simulink model "problem2"  (R2020a)
settings: Solver=VariableStepAuto  StartTime=0.0  StopTime=10.0  RelTol=1e-3
undefined symbols (not defined in the file): be, bv, Ie, Iv, muk, mus, R
settings Model: DataDictionary=variables.sldd  Creator=Jake  LastModifiedBy=Jake
settings SolverCC: ZeroCrossAlgorithm=Adaptive
settings DebuggingCC: IgnoredZcDiagnostic=none

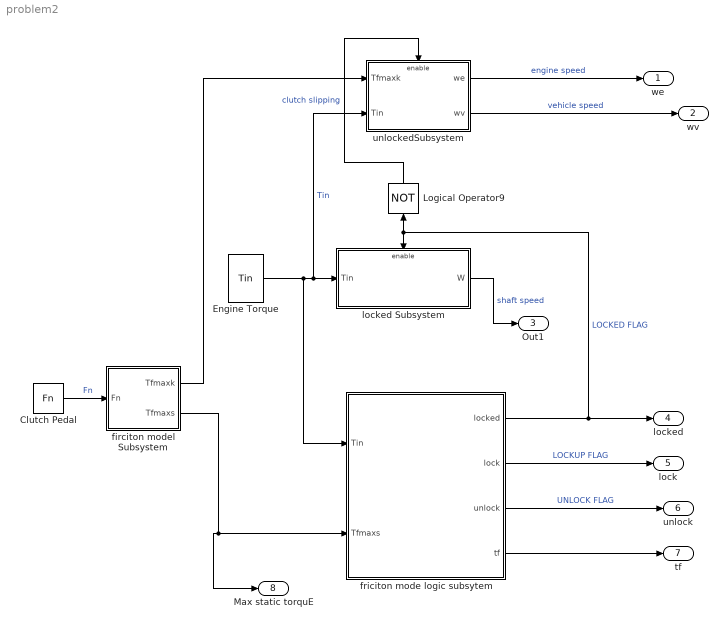
== system problem2 ==
  " firciton model Subsystem" : Subsystem
  " locked Subsystem" : Subsystem
  " unlockedSubsystem" : Subsystem
  Clutch Pedal : FromWorkspace  VariableName=Fn  ZeroCross=off
  Engine Torque : FromWorkspace  VariableName=Tin  ZeroCross=off
  Logical Operator9 : Logic  Operator=NOT  Inputs=1  IconShape=distinctive  OutDataTypeStr=boolean
  friciton mode logic subsytem : Subsystem
  we : Outport
  wv : Outport  Port=2
  Out1 : Outport  Port=3
  locked : Outport  Port=4
  lock : Outport  Port=5
  unlock : Outport  Port=6
  tf : Outport  Port=7
  Max static torquE : Outport  Port=8
  wires:
  " unlockedSubsystem"/1(we) -> we/1  "engine speed"
  " unlockedSubsystem"/2(wv) -> wv/1  "vehicle speed"
  " locked Subsystem"/1(W) -> Out1/1  "shaft speed"
  Engine Torque/1 -> friciton mode logic subsytem/1(Tin), " unlockedSubsystem"/2(Tin), " locked Subsystem"/1(Tin)  "Tin"
  friciton mode logic subsytem/2(lock) -> lock/1  "LOCKUP FLAG"
  friciton mode logic subsytem/3(unlock) -> unlock/1  "UNLOCK FLAG"
  friciton mode logic subsytem/4(tf) -> tf/1
  Logical Operator9/1 -> " unlockedSubsystem"/Enable  "clutch slipping"
  friciton mode logic subsytem/1(locked) -> locked/1, Logical Operator9/1, " locked Subsystem"/Enable  "LOCKED FLAG"
  Clutch Pedal/1 -> " firciton model Subsystem"/1(Fn)  "Fn"
  " firciton model Subsystem"/1(Tfmaxk) -> " unlockedSubsystem"/1(Tfmaxk)
  " firciton model Subsystem"/2(Tfmaxs) -> Max static torquE/1, friciton mode logic subsytem/2(Tfmaxs)

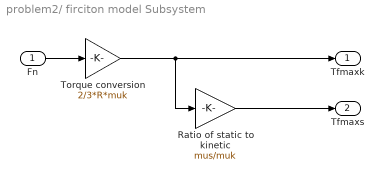
== system problem2/ firciton model Subsystem ==
  Fn : Inport
  Ratio of static to kinetic : Gain  Gain=mus/muk  SaturateOnIntegerOverflow=on  OutDataTypeStr=Inherit: Same as input  ParamDataTypeStr=Inherit: Same as input
  Torque conversion : Gain  Gain=2/3*R*muk  SaturateOnIntegerOverflow=on  OutDataTypeStr=Inherit: Same as input  ParamDataTypeStr=Inherit: Same as input
  Tfmaxk : Outport  InitialOutput=0  VectorParamsAs1DForOutWhenUnconnected=off
  Tfmaxs : Outport  Port=2  InitialOutput=0  VectorParamsAs1DForOutWhenUnconnected=off
  wires:
  Torque conversion/1 -> Tfmaxk/1, Ratio of static to kinetic/1
  Ratio of static to kinetic/1 -> Tfmaxs/1
  Fn/1 -> Torque conversion/1

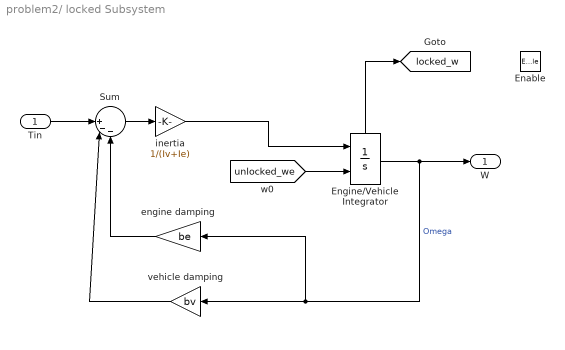
== system problem2/ locked Subsystem ==
  Tin : Inport
  Enable : EnablePort
  Engine/Vehicle Integrator : Integrator  InitialConditionSource=external  ShowStatePort=on
  Sum : Sum  Inputs=||+--  InputSameDT=on  SaturateOnIntegerOverflow=on  OutDataTypeStr=Inherit: Same as first input
  engine damping : Gain  Gain=be
  inertia : Gain  Gain=1/(Iv+Ie)
  vehicle damping : Gain  Gain=bv
  W : Outport
  tag scope: locked_w=global
  wires:
  Engine/Vehicle Integrator/State -> [locked_w]
  Sum/1 -> inertia/1
  Engine/Vehicle Integrator/1 -> W/1, engine damping/1, vehicle damping/1  "Omega"
  inertia/1 -> Engine/Vehicle Integrator/1
  engine damping/1 -> Sum/3
  Tin/1 -> Sum/1
  vehicle damping/1 -> Sum/2
  [unlocked_we] -> Engine/Vehicle Integrator/2

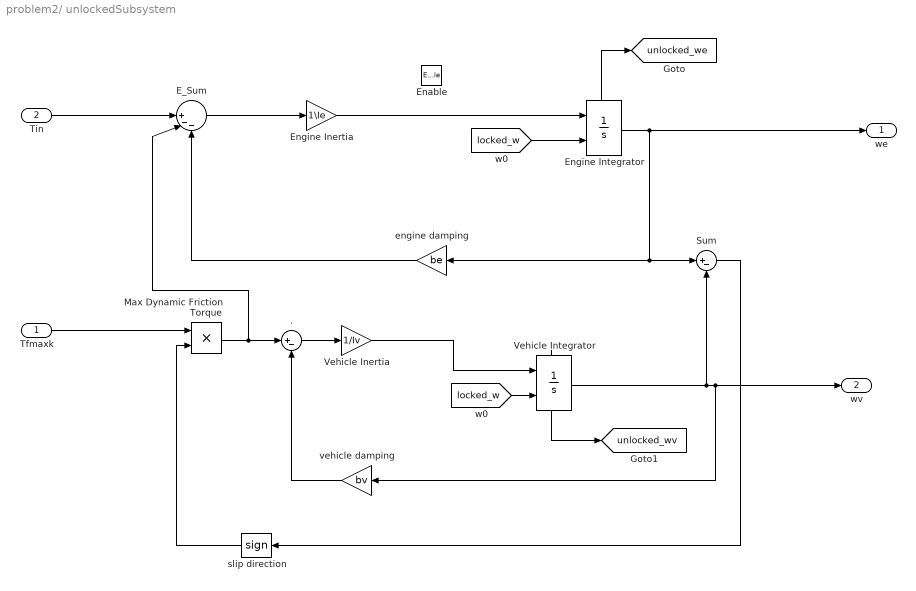
== system problem2/ unlockedSubsystem ==
  Tfmaxk : Inport
  Tin : Inport  Port=2
  Enable : EnablePort
  . : Sum  Inputs=|+-  InputSameDT=on  SaturateOnIntegerOverflow=on  OutDataTypeStr=Inherit: Same as first input
  E_Sum : Sum  Inputs=||+--  InputSameDT=on  SaturateOnIntegerOverflow=on  OutDataTypeStr=Inherit: Same as first input
  Engine Integrator : Integrator  InitialConditionSource=external  ShowStatePort=on
  Engine Inertia : Gain  Gain=1\Ie
  Max Dynamic Friction Torque : Product
  Sum : Sum  Inputs=|+-
  Vehicle Integrator : Integrator  InitialConditionSource=external  ShowStatePort=on
  Vehicle Inertia : Gain  Gain=1/Iv
  engine damping : Gain  Gain=be
  slip direction : Signum
  vehicle damping : Gain  Gain=bv
  we : Outport
  wv : Outport  Port=2
  tag scope: unlocked_we=global, unlocked_wv=global
  wires:
  engine damping/1 -> E_Sum/3
  Engine Integrator/State -> [unlocked_we]
  Engine Integrator/1 -> we/1, engine damping/1, Sum/1
  E_Sum/1 -> Engine Inertia/1
  Max Dynamic Friction Torque/1 -> E_Sum/2, ./1
  slip direction/1 -> Max Dynamic Friction Torque/2
  Tfmaxk/1 -> Max Dynamic Friction Torque/1
  [locked_w] -> Engine Integrator/2
  Vehicle Integrator/1 -> wv/1, vehicle damping/1, Sum/2
  Vehicle Inertia/1 -> Vehicle Integrator/1
  [locked_w] -> Vehicle Integrator/2
  ./1 -> Vehicle Inertia/1
  Vehicle Integrator/State -> [unlocked_wv]
  vehicle damping/1 -> ./2
  Sum/1 -> slip direction/1
  Engine Inertia/1 -> Engine Integrator/1
  Tin/1 -> E_Sum/1

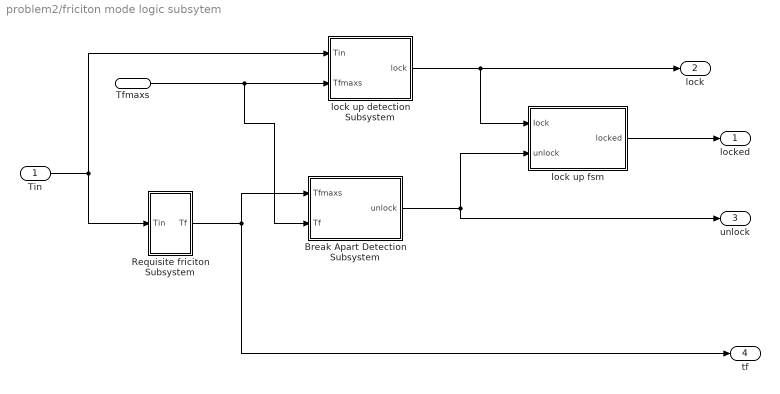
== system problem2/friciton mode logic subsytem ==
  Tin : Inport
  Tfmaxs : Inport  Port=2
  " Requisite friciton Subsystem" : Subsystem
  Break Apart Detection Subsystem : Subsystem
  lock up detection Subsystem : Subsystem
  lock up fsm : Subsystem
  locked : Outport
  lock : Outport  Port=2
  unlock : Outport  Port=3
  tf : Outport  Port=4
  wires:
  lock up fsm/1(locked) -> locked/1
  " Requisite friciton Subsystem"/1(Tf) -> tf/1, Break Apart Detection Subsystem/1(Tfmaxs)
  Tin/1 -> " Requisite friciton Subsystem"/1(Tin), lock up detection Subsystem/1(Tin)
  Break Apart Detection Subsystem/1(unlock) -> unlock/1, lock up fsm/2(unlock)
  lock up detection Subsystem/1(lock) -> lock/1, lock up fsm/1(Iock)
  Tfmaxs/1 -> Break Apart Detection Subsystem/2(Tf), lock up detection Subsystem/2(Tfmaxs)

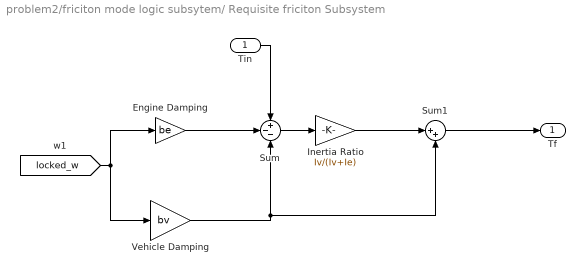
== system problem2/friciton mode logic subsytem/ Requisite friciton Subsystem ==
  Tin : Inport
  Engine Damping : Gain  Gain=be  SaturateOnIntegerOverflow=on  OutDataTypeStr=Inherit: Same as input  ParamDataTypeStr=Inherit: Same as input
  Inertia Ratio : Gain  Gain=Iv/(Iv+Ie)  SaturateOnIntegerOverflow=on  OutDataTypeStr=Inherit: Same as input  ParamDataTypeStr=Inherit: Same as input
  Sum : Sum  Inputs=+--  InputSameDT=on  SaturateOnIntegerOverflow=on  OutDataTypeStr=Inherit: Same as first input
  Sum1 : Sum  Inputs=|++  InputSameDT=on  SaturateOnIntegerOverflow=on  OutDataTypeStr=Inherit: Same as first input
  Vehicle Damping : Gain  Gain=bv  SaturateOnIntegerOverflow=on  OutDataTypeStr=Inherit: Same as input  ParamDataTypeStr=Inherit: Same as input
  Tf : Outport  InitialOutput=0  VectorParamsAs1DForOutWhenUnconnected=off
  wires:
  Sum1/1 -> Tf/1
  [locked_w] -> Vehicle Damping/1, Engine Damping/1
  Tin/1 -> Sum/1
  Vehicle Damping/1 -> Sum/3, Sum1/2
  Engine Damping/1 -> Sum/2
  Sum/1 -> Inertia Ratio/1
  Inertia Ratio/1 -> Sum1/1

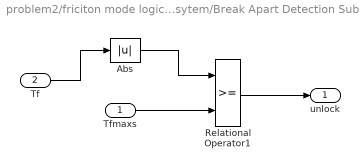
== system problem2/friciton mode logic subsytem/Break Apart Detection Subsystem ==
  Tfmaxs : Inport
  Tf : Inport  Port=2
  Abs : Abs  SaturateOnIntegerOverflow=on
  Relational Operator1 : RelationalOperator  OutDataTypeStr=boolean  RndMeth=Nearest  InputSameDT=on
  unlock : Outport
  wires:
  Tfmaxs/1 -> Relational Operator1/2
  Abs/1 -> Relational Operator1/1
  Relational Operator1/1 -> unlock/1
  Tf/1 -> Abs/1

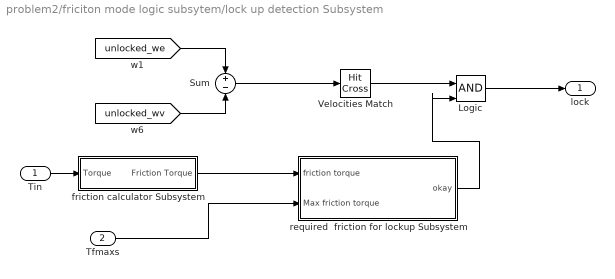
== system problem2/friciton mode logic subsytem/lock up detection Subsystem ==
  Tin : Inport
  Tfmaxs : Inport  Port=2
  " friction calculator Subsystem" : Subsystem
  " required  friction for lockup Subsystem" : Subsystem
  Logic : Logic  IconShape=distinctive  OutDataTypeStr=boolean
  Sum : Sum  Inputs=+-  InputSameDT=on  SaturateOnIntegerOverflow=on  OutDataTypeStr=Inherit: Same as first input
  Velocities Match : HitCross
  lock : Outport
  wires:
  Logic/1 -> lock/1
  [unlocked_we] -> Sum/1
  " required  friction for lockup Subsystem"/1(okay) -> Logic/2
  Velocities Match/1 -> Logic/1
  [unlocked_wv] -> Sum/2
  Tin/1 -> " friction calculator Subsystem"/1(Torque)
  Tfmaxs/1 -> " required  friction for lockup Subsystem"/2(Max friction torque)
  " friction calculator Subsystem"/1(Friction Torque) -> " required  friction for lockup Subsystem"/1(friction torque)
  Sum/1 -> Velocities Match/1

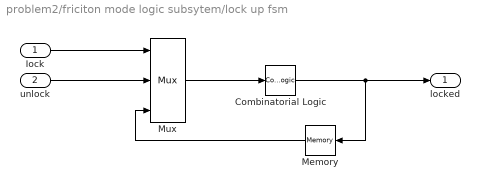
== system problem2/friciton mode logic subsytem/lock up fsm ==
  Iock : Inport
  unlock : Inport  Port=2
  Combinatorial Logic : CombinatorialLogic  TruthTable=[0;1;0;0;1;1;1;0]
  Memory : Memory
  Mux : Mux  Inputs=3
  locked : Outport
  wires:
  Memory/1 -> Mux/3
  Combinatorial Logic/1 -> locked/1, Memory/1
  Mux/1 -> Combinatorial Logic/1
  unlock/1 -> Mux/2
  Iock/1 -> Mux/1

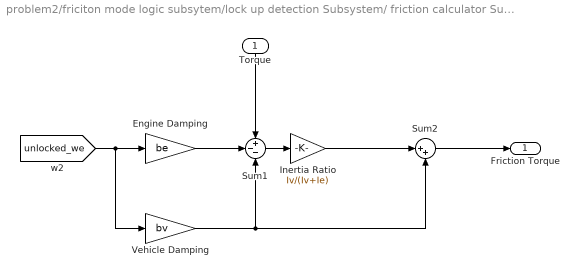
== system problem2/friciton mode logic subsytem/lock up detection Subsystem/ friction calculator Subsystem ==
  Torque : Inport
  Engine Damping : Gain  Gain=be  SaturateOnIntegerOverflow=on  OutDataTypeStr=Inherit: Same as input  ParamDataTypeStr=Inherit: Same as input
  Inertia Ratio : Gain  Gain=Iv/(Iv+Ie)  SaturateOnIntegerOverflow=on  OutDataTypeStr=Inherit: Same as input  ParamDataTypeStr=Inherit: Same as input
  Sum1 : Sum  Inputs=+--  InputSameDT=on  SaturateOnIntegerOverflow=on  OutDataTypeStr=Inherit: Same as first input
  Sum2 : Sum  Inputs=|++  InputSameDT=on  SaturateOnIntegerOverflow=on  OutDataTypeStr=Inherit: Same as first input
  Vehicle Damping : Gain  Gain=bv  SaturateOnIntegerOverflow=on  OutDataTypeStr=Inherit: Same as input  ParamDataTypeStr=Inherit: Same as input
  Friction Torque : Outport  InitialOutput=0  VectorParamsAs1DForOutWhenUnconnected=off
  wires:
  Engine Damping/1 -> Sum1/2
  [unlocked_we] -> Vehicle Damping/1, Engine Damping/1
  Vehicle Damping/1 -> Sum2/2, Sum1/3
  Inertia Ratio/1 -> Sum2/1
  Sum2/1 -> Friction Torque/1
  Sum1/1 -> Inertia Ratio/1
  Torque/1 -> Sum1/1

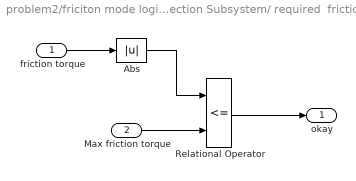
== system problem2/friciton mode logic subsytem/lock up detection Subsystem/ required  friction for lockup Subsystem ==
  friction torque : Inport
  Max friction torque : Inport  Port=2
  Abs : Abs  SaturateOnIntegerOverflow=on
  Relational Operator : RelationalOperator  Operator=<=  OutDataTypeStr=boolean  RndMeth=Nearest  InputSameDT=on
  okay : Outport
  wires:
  Max friction torque/1 -> Relational Operator/2
  Abs/1 -> Relational Operator/1
  Relational Operator/1 -> okay/1
  friction torque/1 -> Abs/1
